simulink model "equation_modelling"  (R2025a)
settings: Solver=FixedStepAuto  StartTime=0.0  StopTime=100.0  RelTol=1e-3
settings Model: Creator=Kush  LastModifiedBy=Kush
settings OptimizationCC: DefaultParameterBehavior=Inlined  EnhancedBackFolding=on  PassReuseOutputArgsAs=Individual arguments  ZeroExternalMemoryAtStartup=off  ZeroInternalMemoryAtStartup=off  MaxStackSize=64  OptimizeBlockOrder=speed  DifferentSizesBufferReuse=on  OptimizationCustomize=off  EfficientTunableParamExpr=on
settings DebuggingCC: ParameterTunabilityLossMsg=error
settings SFSimCC: MATLABDynamicMemAlloc=off
settings RTWCC: SystemTargetFile=ert.tlc  HardwareBoard=Robot Operating System 2 (ROS 2)  TLCOptions="-aInlineSetEventsForThisBaseRateFcn=TLC_FALSE -aSuppressMultiTaskScheduler=TLC_FALSE  -aRateBasedStepFcn=0"  TemplateMakefile=ert_default_tmf  Toolchain=Colcon Tools  TargetLang=C++  Description=Embedded Coder
settings CodeAppCC: ForceParamTrailComments=on  IgnoreCustomStorageClasses=off  OperatorAnnotations=on  SimulinkDataObjDesc=on  SFDataObjDesc=on  InsertBlockDesc=on
settings ERTTargetCC: ExtModeTransport=2.0  RootIOFormat=Structure reference  CodeInterfacePackaging=C++ class

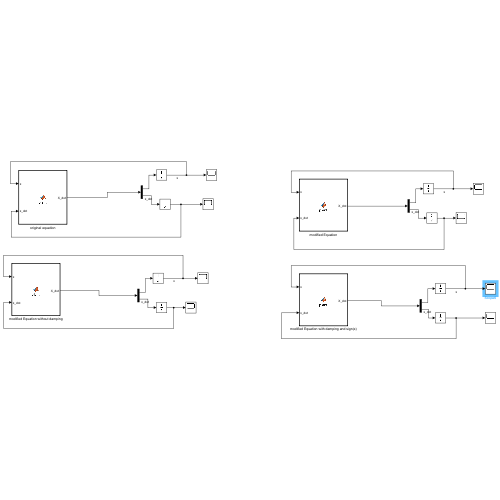
[thumbnail: Simulink's stored preview of the top-level diagram]
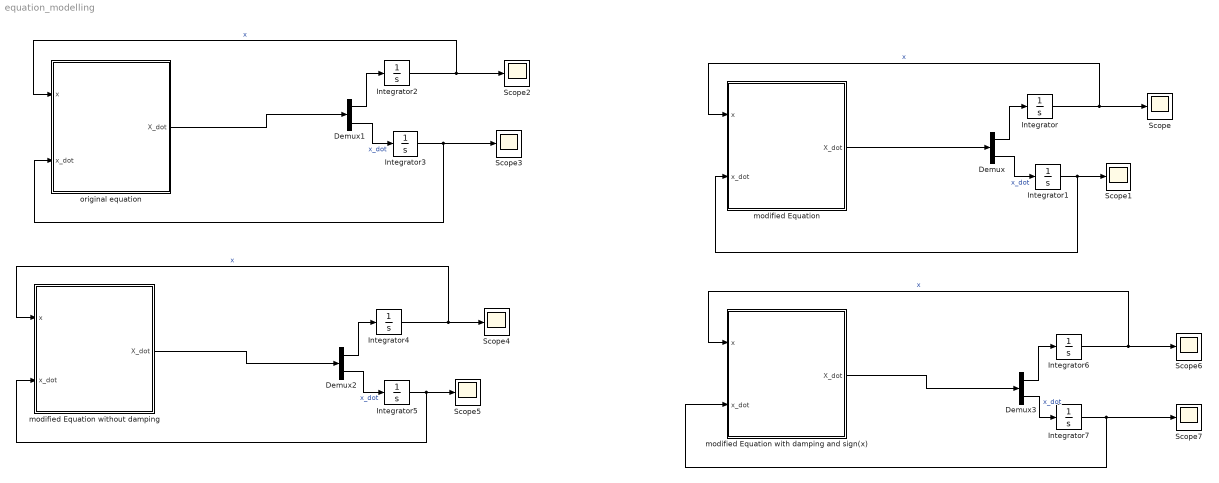
== system equation_modelling ==
  Demux{,1..3} (4 alike) : Demux  Outputs=2
  Integrator{,2,4,6} (4 alike) : Integrator
  Integrator{1,3,5,7} (4 alike) : Integrator  InitialCondition=0.5
  Scope{,1..7} (8 alike) : Scope
      Scope settings: ActiveDisplayYMinimum=-1.5713145837821652  ActiveDisplayYMaximum=2.3070195658216757
      Scope1 settings: ActiveDisplayYMinimum=-1  ActiveDisplayYMaximum=1
      Scope2 settings: SampleTime=0.001  ActiveDisplayYMinimum=-1.7504309440804662  ActiveDisplayYMaximum=1.2752780790586884  DataLoggingVariableName=ScopeData2
      Scope3 settings: ActiveDisplayYMinimum=-0.69315005082747594  ActiveDisplayYMaximum=0.69492143715181309  DataLoggingVariableName=ScopeData3
      Scope4 settings: ActiveDisplayYMinimum=-1.5999407190127664  ActiveDisplayYMaximum=15.381792482722576  DataLoggingVariableName=ScopeData4
      Scope5 settings: ActiveDisplayYMinimum=-42439.282136972783  ActiveDisplayYMaximum=381955.79491573491  DataLoggingVariableName=ScopeData5
      Scope6 settings: ActiveDisplayYMinimum=-1.5464942332147824  ActiveDisplayYMaximum=1.2774815378814572  DataLoggingVariableName=ScopeData6
      Scope7 settings: ActiveDisplayYMinimum=-1  ActiveDisplayYMaximum=1  DataLoggingVariableName=ScopeData7
  modified Equation : MATLAB Function  TreatAsAtomicUnit=on
  modified Equation with damping and sign(x) : MATLAB Function  TreatAsAtomicUnit=on
  modified Equation without damping : MATLAB Function  TreatAsAtomicUnit=on
  original equation : MATLAB Function  TreatAsAtomicUnit=on
  wires:
  modified Equation/1(X_dot) -> Demux/1
  Demux/1 -> Integrator/1
  Integrator/1 -> modified Equation/1(x), Scope/1  "x"
  Demux/2 -> Integrator1/1  "x_dot"
  Integrator1/1 -> modified Equation/2(x_dot), Scope1/1
  Integrator2/1 -> original equation/1(x), Scope2/1  "x"
  Demux1/1 -> Integrator2/1
  Integrator3/1 -> original equation/2(x_dot), Scope3/1
  original equation/1(X_dot) -> Demux1/1
  Demux1/2 -> Integrator3/1  "x_dot"
  Integrator4/1 -> modified Equation without damping/1(x), Scope4/1  "x"
  Demux2/1 -> Integrator4/1
  Integrator5/1 -> modified Equation without damping/2(x_dot), Scope5/1
  modified Equation without damping/1(X_dot) -> Demux2/1
  Demux2/2 -> Integrator5/1  "x_dot"
  Demux3/1 -> Integrator6/1
  Integrator7/1 -> modified Equation with damping and sign(x)/2(x_dot), Scope7/1
  modified Equation with damping and sign(x)/1(X_dot) -> Demux3/1
  Integrator6/1 -> modified Equation with damping and sign(x)/1(x), Scope6/1  "x"
  Demux3/2 -> Integrator7/1  "x_dot"

== matlab function equation_modelling/original equation ==
  data: x input; X_dot output; x_dot input
function X_dot = plant(x, x_dot)
% Parameters
k = 1;
L = 0.5;
A = 1;
B = 5;


if abs(x) >= L
    x = sign(x) * (L - 1e-6);
end

den = 1 - abs(x)/L;
u = k * sign(x) .* log(den);

x_ddot = u;
X_dot = [x_dot; x_ddot];
end

== matlab function equation_modelling/modified Equation ==
  data: x input; x_dot input; X_dot output
function X_dot = plant(x, x_dot)
% Parameters
k = 1;
L = 0.5;
A = 1;
B = 5;


den = 1 - abs(x)/L;
if abs(den) < 1e-6
    den = sign(den)*1e-6;
end

arg = B / den;
u = -k * x * sqrt(abs(x)/L) * tanh(arg) - A * x_dot;

x_ddot = u;
X_dot = [x_dot; x_ddot];
end

== matlab function equation_modelling/modified Equation without damping ==
  data: x input; x_dot input; X_dot output
function X_dot = plant(x, x_dot)
% Parameters
k = 1;
L = 0.5;
A = 1;
B = 5;


den = 1 - abs(x)/L;
if abs(den) < 1e-6
    den = sign(den)*1e-6;
end

arg = B / den;
u = -k * x * sqrt(abs(x)/L) * tanh(arg);

x_ddot = u;
X_dot = [x_dot; x_ddot];
end

== matlab function equation_modelling/modified Equation with damping and sign(x) ==
  data: x input; x_dot input; X_dot output
function X_dot = plant(x, x_dot)
% Parameters
k = 1;
L = 0.5;
A = 1;
B = 5;


den = 1 - abs(x)/L;
if abs(den) < 1e-6
    den = sign(den)*1e-6;
end

arg = B / den;
u = -k * sign(x) * sqrt(abs(x)/L) * tanh(arg) -A*x_dot;

x_ddot = u;
X_dot = [x_dot; x_ddot];
end
